simulink model "DESHAN_2022E039_LAB04_1"  (R2024a)
settings: Solver=VariableStepAuto  StartTime=0.0  StopTime=0.1  RelTol=1e-3
settings Model: Creator=dcrea  LastModifiedBy=dcrea

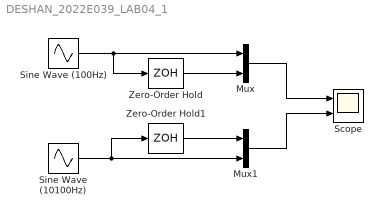
== system DESHAN_2022E039_LAB04_1 ==
  Mux : Mux  Inputs=2
  Mux1 : Mux  Inputs=2
  Scope : Scope  NumInputPorts=2
  Sine Wave (100Hz) : Sin  Frequency=100  SampleTime=0
  Sine Wave (10100Hz) : Sin  Frequency=9900  SampleTime=0
  Zero-Order Hold : ZeroOrderHold  SampleTime=0.0001
  Zero-Order Hold1 : ZeroOrderHold  SampleTime=0.0001
  wires:
  Sine Wave (100Hz)/1 -> Zero-Order Hold/1, Mux/1
  Sine Wave (10100Hz)/1 -> Mux1/2, Zero-Order Hold1/1
  Zero-Order Hold/1 -> Mux/2
  Zero-Order Hold1/1 -> Mux1/1
  Mux/1 -> Scope/1
  Mux1/1 -> Scope/2
